simulink model "VB_RI_EKF_GNSS_INS25"  (R2023a)
settings: Solver=FixedStepAuto  StartTime=0  StopTime=200  FixedStep=0.01  RelTol=1e-3
InitFcn:
  | %resilient_initNavigation1216;
  | %init_param;
values from neighbouring files (symbols this model uses):
  C = zeros(n,m)    [utchol.m]
undefined symbols (not defined in the file or in its folder): dt, dtDelay, g0, gam0_rad, GNSSoutragetime, ISUS_flag, magnitude, p, P0, P0_RIEKF, param, pd0, pe0, phi0_rad, pn0, psi, psi0_rad, state_dim, vd0, ve0, vn0
libraries: simulink_extras x133, simulink x81, dspstat3 x81, sharedtransform x69, sharedTrackingLibrary x17, matrix_library x15, deeplib x6, dspfactors x4, aerolibconvert2 x4, aerolibtransform2 x4, dspsrcs4 x1
(part 24 of 32)

== system VB_RI_EKF_GNSS_INS25/ISUS_RIEKF3/Error State Kalman Filter M2/Extended Kalman Filter M1/Predict/If Action Subsystem ==
  Action Port : ActionPort
  Constant : Constant  Value=0
  Data Store Read : DataStoreRead  DataStoreName=x  IndexOptions=Index vector (dialog)  Indices=1  OutputSizes=1
  Data Store Write : DataStoreWrite  DataStoreName=x  IndexOptions=Index vector (dialog)  Indices=1  OutputSizes=1
  Data Store Write1 : DataStoreWrite  DataStoreName=feedback_flag_18dim  IndexOptions=Index vector (dialog)  Indices=1  OutputSizes=1
  Mux : Mux  Inputs=2
  Selector : Selector  InputPortWidth=18  IndexOptions=Index vector (dialog)  Indices=[16 17 18]  OutputSizes=1
  Zero : Constant  Value=zeros(15,1)  OutDataTypeStr=Inherit: Inherit via back propagation
  wires:
  Mux/1 -> Data Store Write/1
  Selector/1 -> Mux/2
  Zero/1 -> Mux/1
  Data Store Read/1 -> Selector/1
  Constant/1 -> Data Store Write1/1

== system VB_RI_EKF_GNSS_INS25/ISUS_RIEKF3/Error State Kalman Filter M2/bak/Simulink Function - State Transition Jacobian/Cal Phi1 ==
  Rbn : Inport
  vn : Inport  Port=2
  pn : Inport  Port=3
  Constant : Constant  Value=dt
  MATLAB Function1 : MATLAB Function  TreatAsAtomicUnit=on
  Reshape : Reshape  OutputDimensionality=Column vector (2-D)
  Reshape1 : Reshape  OutputDimensionality=Column vector (2-D)
  Phi : Outport
  wires:
  Constant/1 -> MATLAB Function1/4(dt)
  MATLAB Function1/1(Phi) -> Phi/1
  Rbn/1 -> MATLAB Function1/3(Rbn)
  vn/1 -> Reshape/1
  pn/1 -> Reshape1/1
  Reshape/1 -> MATLAB Function1/1(vn)
  Reshape1/1 -> MATLAB Function1/2(pn)

== system VB_RI_EKF_GNSS_INS25/ISUS_RIEKF3/Error State Kalman Filter M3/Extended Kalman Filter M1/Correct M1/Subsystem2 ==
  Pk_1_ISIU : Inport
  Pk_2 : Inport  Port=2
  Constant : Constant  Value=ISUS_flag
  Data Type Conversion : DataTypeConversion  OutDataTypeStr=single  SaturateOnIntegerOverflow=off  RndMeth=Floor
  MATLAB Function1 : MATLAB Function  TreatAsAtomicUnit=on
  y1 : Outport
  wires:
  MATLAB Function1/1(y) -> y1/1
  Pk_1_ISIU/1 -> Data Type Conversion/1
  Pk_2/1 -> MATLAB Function1/2(X)
  Constant/1 -> MATLAB Function1/3(ISUS_flag)
  Data Type Conversion/1 -> MATLAB Function1/1(u)

== system VB_RI_EKF_GNSS_INS25/ISUS_RIEKF3/Error State Kalman Filter M3/Extended Kalman Filter M1/Correct M1/innovation calculation1 ==
  Pk/k_1 : Inport
  yMeas : Inport  Port=2
  X : Inport  Port=3
  R : Inport  Port=4
  H : Inport  Port=5
  beta_k : Inport  Port=6
  Rk1 : Inport  Port=7
  Add : Sum
  Add1 : Sum  Inputs=+-
  Cast To Double1 : DataTypeConversion  OutDataTypeStr=single  SaturateOnIntegerOverflow=off  RndMeth=Floor
  Cast To Double2 : DataTypeConversion  OutDataTypeStr=single  SaturateOnIntegerOverflow=off  RndMeth=Floor
  Constant : Constant  Value=1/3  OutDataTypeStr=single
  Delay : Delay  DelayLength=1  InitialConditionSource=Input port
      settings: InputPortMap=u0,p4
  MATLAB Function : MATLAB Function  TreatAsAtomicUnit=on
  MATLAB Function1 : MATLAB Function  TreatAsAtomicUnit=on
  MATLAB Function2 : MATLAB Function  TreatAsAtomicUnit=on
  MATLAB Function4 : MATLAB Function  Commented=on  TreatAsAtomicUnit=on
  Product : Product  Inputs=3  Multiplication=Matrix(*)
  Product1 : Product  Multiplication=Matrix(*)
  Product2 : Product  Multiplication=Matrix(*)
  Scope1 : Scope
  Scope2 : Scope
  Transpose : Math  Operator=transpose
  Transpose1 : Math  Operator=transpose
  Sk : Outport
  m_innov : Outport  Port=2
  beta : Outport  Port=3
  R_k : Outport  Port=4
  wires:
  MATLAB Function/1(y) -> Product/2
  Product/1 -> Add/1
  Transpose/1 -> Product/3
  R/1 -> MATLAB Function2/2(R)
  Pk/k_1/1 -> MATLAB Function/1(u)
  yMeas/1 -> Add1/1
  H/1 -> Product1/1, Product/1, Transpose/1
  X/1 -> Product1/2, Scope2/1
  Product1/1 -> Add1/2
  Add/1 -> Cast To Double1/1  "S"
  Add1/1 -> Product2/2, Transpose1/1, m_innov/1, Scope1/1
  Transpose1/1 -> Product2/1
  MATLAB Function2/1(R_k) -> Cast To Double2/1
  beta_k/1 -> Delay/1
  Constant/1 -> Delay/2
  Delay/1 -> MATLAB Function2/1(beta_k)
  MATLAB Function1/1(beta) -> beta/1
  Cast To Double1/1 -> MATLAB Function1/2(S), Sk/1
  Cast To Double2/1 -> R_k/1
  Rk1/1 -> Add/2
  Product2/1 -> MATLAB Function1/1(r)

== system VB_RI_EKF_GNSS_INS25/ISUS_RIEKF3/Error State Kalman Filter M3/Extended Kalman Filter M1/Predict/If Action Subsystem ==
  Action Port : ActionPort
  Constant : Constant  Value=0
  Data Store Read : DataStoreRead  DataStoreName=x  IndexOptions=Index vector (dialog)  Indices=1  OutputSizes=1
  Data Store Write : DataStoreWrite  DataStoreName=x  IndexOptions=Index vector (dialog)  Indices=1  OutputSizes=1
  Data Store Write1 : DataStoreWrite  DataStoreName=feedback_flag_18dim  IndexOptions=Index vector (dialog)  Indices=1  OutputSizes=1
  Mux : Mux  Inputs=2
  Selector : Selector  InputPortWidth=18  IndexOptions=Index vector (dialog)  Indices=[16 17 18]  OutputSizes=1
  Zero : Constant  Value=zeros(15,1)  OutDataTypeStr=Inherit: Inherit via back propagation
  wires:
  Constant/1 -> Data Store Write1/1
  Data Store Read/1 -> Selector/1
  Zero/1 -> Mux/1
  Selector/1 -> Mux/2
  Mux/1 -> Data Store Write/1

== system VB_RI_EKF_GNSS_INS25/ISUS_RIEKF3/Error State Kalman Filter M3/bak/Simulink Function - State Transition Jacobian/Cal Phi1 ==
  Rbn : Inport
  vn : Inport  Port=2
  pn : Inport  Port=3
  Constant : Constant  Value=dt
  MATLAB Function1 : MATLAB Function  TreatAsAtomicUnit=on
  Reshape : Reshape  OutputDimensionality=Column vector (2-D)
  Reshape1 : Reshape  OutputDimensionality=Column vector (2-D)
  Phi : Outport
  wires:
  Reshape1/1 -> MATLAB Function1/2(pn)
  Reshape/1 -> MATLAB Function1/1(vn)
  pn/1 -> Reshape1/1
  vn/1 -> Reshape/1
  Rbn/1 -> MATLAB Function1/3(Rbn)
  MATLAB Function1/1(Phi) -> Phi/1
  Constant/1 -> MATLAB Function1/4(dt)

== system VB_RI_EKF_GNSS_INS25/ISUS_RIEKF3/INS propogation/Init_PVQ/Horizontal_attitude/Deal with zero ==
  In1 : Inport
  Add5 : Sum
  Constant1 : Constant  Value=1e-6  OutDataTypeStr=single
  Out1 : Outport
  wires:
  Constant1/1 -> Add5/2
  In1/1 -> Add5/1
  Add5/1 -> Out1/1

== system VB_RI_EKF_GNSS_INS25/ISUS_RIEKF3/INS propogation/gyro bias compensation/error compensation/If Action Subsystem1 ==
  Action Port : ActionPort  ActionPortLabel=if(u1 == 1)
  Constant : Constant
  Data Store Write : DataStoreWrite  DataStoreName=feedback_flag_18dim_RIEKF  IndexOptions=Index vector (dialog)  Indices=1  OutputSizes=1
  wires:
  Constant/1 -> Data Store Write/1

== system VB_RI_EKF_GNSS_INS25/ISUS_RIEKF3/INS propogation1/Init_PVQ/Horizontal_attitude/Deal with zero ==
  In1 : Inport
  Add5 : Sum
  Constant1 : Constant  Value=1e-6  OutDataTypeStr=single
  Out1 : Outport
  wires:
  Add5/1 -> Out1/1
  In1/1 -> Add5/1
  Constant1/1 -> Add5/2

== system VB_RI_EKF_GNSS_INS25/ISUS_RIEKF3/INS propogation1/gyro bias compensation/error compensation/If Action Subsystem1 ==
  Action Port : ActionPort  ActionPortLabel=if(u1 == 1)
  Constant : Constant
  Data Store Write : DataStoreWrite  DataStoreName=feedback_flag_18dim_RIEKF  IndexOptions=Index vector (dialog)  Indices=1  OutputSizes=1
  wires:
  Constant/1 -> Data Store Write/1

== system VB_RI_EKF_GNSS_INS25/ISUS_RIEKF3/INS propogation2/Init_PVQ/Horizontal_attitude/Deal with zero ==
  In1 : Inport
  Add5 : Sum
  Constant1 : Constant  Value=1e-6  OutDataTypeStr=single
  Out1 : Outport
  wires:
  Constant1/1 -> Add5/2
  In1/1 -> Add5/1
  Add5/1 -> Out1/1

== system VB_RI_EKF_GNSS_INS25/ISUS_RIEKF3/INS propogation2/gyro bias compensation/error compensation/If Action Subsystem1 ==
  Action Port : ActionPort  ActionPortLabel=if(u1 == 1)
  Constant : Constant
  Data Store Write : DataStoreWrite  DataStoreName=feedback_flag_18dim_RIEKF  IndexOptions=Index vector (dialog)  Indices=1  OutputSizes=1
  wires:
  Constant/1 -> Data Store Write/1

== system VB_RI_EKF_GNSS_INS25/ISUS_RIEKF3/INS propogation3/Init_PVQ/Horizontal_attitude/Deal with zero ==
  In1 : Inport
  Add5 : Sum
  Constant1 : Constant  Value=1e-6  OutDataTypeStr=single
  Out1 : Outport
  wires:
  Add5/1 -> Out1/1
  In1/1 -> Add5/1
  Constant1/1 -> Add5/2

== system VB_RI_EKF_GNSS_INS25/ISUS_RIEKF3/INS propogation3/gyro bias compensation/error compensation/If Action Subsystem1 ==
  Action Port : ActionPort  ActionPortLabel=if(u1 == 1)
  Constant : Constant
  Data Store Write : DataStoreWrite  DataStoreName=feedback_flag_18dim_RIEKF  IndexOptions=Index vector (dialog)  Indices=1  OutputSizes=1
  wires:
  Constant/1 -> Data Store Write/1

== system VB_RI_EKF_GNSS_INS25/RI EKF_AOA_LSTM/Error State Kalman Filter/Extended Kalman Filter1/Correct1/IGG_check ==
  Pk/k_1 : Inport
  yMeas : Inport  Port=2
  X : Inport  Port=3
  R : Inport  Port=4
  Abs : Abs  Commented=on  SaturateOnIntegerOverflow=off
  Abs1 : Abs  Commented=on  SaturateOnIntegerOverflow=off
  Add : Sum  Commented=on
  Add1 : Sum  Inputs=+-
  Add2 : Sum  Commented=on
  Constant : Constant  Commented=on  Value=12
  Constant1 : Constant  Commented=on  Value=8
  Constant2 : Constant  Value=25
  Constant3 : Constant  Commented=on  Value=eps
  Constant4 : Constant  Commented=on  Value=15
  Constant6 : Constant  Value=[zeros(6,3),eye(6),zeros(6,6)]  OutDataTypeStr=single
  Divide : Product  Commented=on  Inputs=*/
  Extract Diagonal1 : matrix_library/Extract Diagonal  Commented=on
  MATLAB Function : MATLAB Function  Commented=on  TreatAsAtomicUnit=on
  Product : Product  Inputs=3  Multiplication=Matrix(*)
  Product1 : Product  Multiplication=Matrix(*)
  Product2 : Product
  Scope : Scope  Commented=on
  Sqrt1 : Sqrt  Commented=on
  Transpose : Math  Operator=transpose
  yMeas1 : InportShadow  Port=2
  yMeas_out : Outport
  w : Outport  Port=2
  inno : Outport  Port=3
  wires:
  Product/1 -> Add/1
  Transpose/1 -> Product/3
  R/1 -> Add/2
  Pk/k_1/1 -> Product/2
  yMeas/1 -> Add1/1
  Constant6/1 -> Product1/1, Product/1, Transpose/1
  X/1 -> Product1/2
  Product1/1 -> Add1/2
  Product2/1 -> yMeas_out/1
  Add/1 -> Extract Diagonal1/1  "S"
  Divide/1 -> Abs/1, Scope/1
  MATLAB Function/1(w) -> w/1, Product2/1
  Extract Diagonal1/1 -> Abs1/1
  Add1/1 -> inno/1, Divide/1
  Sqrt1/1 -> Add2/1
  Abs/1 -> MATLAB Function/1(err)
  Abs1/1 -> Sqrt1/1
  Add2/1 -> Divide/2
  Constant3/1 -> Add2/2
  yMeas1/1 -> Product2/2
  Constant1/1 -> MATLAB Function/2(k0)
  Constant4/1 -> MATLAB Function/3(k1)
  Constant/1 -> MATLAB Function/4(zk0)
  Constant2/1 -> MATLAB Function/5(zk1)

== system VB_RI_EKF_GNSS_INS25/RI EKF_AOA_LSTM/Error State Kalman Filter/Extended Kalman Filter1/Predict/If Action Subsystem ==
  Action Port : ActionPort
  Constant : Constant  Value=0
  Data Store Read : DataStoreRead  DataStoreName=x  IndexOptions=Index vector (dialog)  Indices=1  OutputSizes=1
  Data Store Write : DataStoreWrite  DataStoreName=x  IndexOptions=Index vector (dialog)  Indices=1  OutputSizes=1
  Data Store Write1 : DataStoreWrite  DataStoreName=feedback_flag_18dim  IndexOptions=Index vector (dialog)  Indices=1  OutputSizes=1
  Mux : Mux  Inputs=2
  Selector : Selector  InputPortWidth=18  IndexOptions=Index vector (dialog)  Indices=[16 17 18]  OutputSizes=1
  Zero : Constant  Value=zeros(15,1)  OutDataTypeStr=Inherit: Inherit via back propagation
  wires:
  Mux/1 -> Data Store Write/1
  Selector/1 -> Mux/2
  Zero/1 -> Mux/1
  Data Store Read/1 -> Selector/1
  Constant/1 -> Data Store Write1/1

== system VB_RI_EKF_GNSS_INS25/RI EKF_AOA_LSTM/Error State Kalman Filter/bak/Simulink Function - State Transition Jacobian/Cal Phi1 ==
  Rbn : Inport
  vn : Inport  Port=2
  pn : Inport  Port=3
  Constant : Constant  Value=dt
  MATLAB Function1 : MATLAB Function  TreatAsAtomicUnit=on
  Reshape : Reshape  OutputDimensionality=Column vector (2-D)
  Reshape1 : Reshape  OutputDimensionality=Column vector (2-D)
  Phi : Outport
  wires:
  Constant/1 -> MATLAB Function1/4(dt)
  MATLAB Function1/1(Phi) -> Phi/1
  Rbn/1 -> MATLAB Function1/3(Rbn)
  vn/1 -> Reshape/1
  pn/1 -> Reshape1/1
  Reshape/1 -> MATLAB Function1/1(vn)
  Reshape1/1 -> MATLAB Function1/2(pn)

== system VB_RI_EKF_GNSS_INS25/RI EKF_AOA_LSTM/INS propogation/AOA//SA//Vwind update/Subsystem/Subsystem ==
  In1 : Inport
  v : Inport  Port=2
  Asin : Trigonometry  Operator=asin
  Math Function : Math  Operator=magnitude^2
  Product1 : Product
  Reciprocal Sqrt : Sqrt  Operator=rSqrt
  Sum of Elements : Sum  Inputs=+
  beta : Outport
  wires:
  Product1/1 -> Asin/1
  Sum of Elements/1 -> Reciprocal Sqrt/1
  Math Function/1 -> Sum of Elements/1
  Reciprocal Sqrt/1 -> Product1/1
  Asin/1 -> beta/1  "beta"
  In1/1 -> Math Function/1
  v/1 -> Product1/2

== system VB_RI_EKF_GNSS_INS25/RI EKF_AOA_LSTM/INS propogation/AOA//SA//Vwind update/Subsystem/Subsystem1 ==
  gyro_raw : Inport
  elevator_aileron_rudder_deg : Inport  Port=2
  accl_raw : Inport  Port=3
  TAS : Inport  Port=4
  Enable : EnablePort
  Compare To Constant : simulink/Logic and Bit Operations/Compare To Constant  relop===  const=9  OutDataTypeStr=boolean
  Counter Limited : simulink/Sources/Counter Limited  uplimit=9  tsamp=-1
  Data Type Conversion5 : DataTypeConversion  OutDataTypeStr=single  SaturateOnIntegerOverflow=off  RndMeth=Floor
  Degrees to Radians{,1..5} (6 alike) : simulink_extras/Transformations/Degrees to Radians
  LSTM predict : Subsystem
  LSTM predict1 : Subsystem
  MATLAB Function1 : MATLAB Function  TreatAsAtomicUnit=on
  MATLAB Function3 : MATLAB Function  TreatAsAtomicUnit=on
  MATLAB Function4 : MATLAB Function  Commented=on  TreatAsAtomicUnit=on
  Memory : Memory
  Memory1 : Memory
  Moving Average1 : dspstat3/Moving Average  Method=Sliding window  ForgettingFactorPort=off  SpecifyWindowLength=on  WindowLength=4  OverlapLength=3  AllowArbitraryInputLength=off  ForgettingFactor=0.9  SimulateUsing=Code generation
  Mux : Mux  Inputs=3
  Mux1 : Mux
  Radians to Degrees5 : simulink_extras/Transformations/Radians to Degrees  Commented=on
  Scope : Scope
  Selector : Selector  InputPortWidth=3  IndexOptions=Index vector (dialog)  Indices=[2]  OutputSizes=1
  Selector{1..3,5} (4 alike) : Selector  InputPortWidth=3  IndexOptions=Index vector (dialog)  Indices=[1]  OutputSizes=1
  Selector4 : Selector  InputPortWidth=3  IndexOptions=Index vector (dialog)  Indices=[3]  OutputSizes=1
  Selector6 : Selector  InputPortWidth=3  IndexOptions=Index vector (dialog)  Indices=[3]  OutputSizes=1
  TAS_1 : InportShadow  Port=4
  az : InportShadow  Port=3
  elevator_aileron_rudder_deg_1 : InportShadow  Port=2
  gyro_raw_1 : InportShadow
  AOA_LSTM_rad out : Outport
  SA_LSTM_rad : Outport  Port=2
  wires:
  elevator_aileron_rudder_deg_1/1 -> Selector6/1
  TAS/1 -> Selector2/1
  gyro_raw/1 -> Selector/1
  Degrees to Radians5/1 -> SA_LSTM_rad/1
  Degrees to Radians/1 -> Mux/3
  Selector1/1 -> Degrees to Radians/1
  Memory1/1 -> MATLAB Function3/4(beta)
  MATLAB Function1/1(Cl) -> Data Type Conversion5/1
  accl_raw/1 -> MATLAB Function1/1(axyz)
  Mux/1 -> LSTM predict/1(X), MATLAB Function4/1(u)
  MATLAB Function3/1(Cy) -> Mux1/2
  Selector/1 -> Mux/1
  Selector2/1 -> MATLAB Function1/2(TAS)  "|TAS|"
  LSTM predict1/1(YPred_test_out) -> Degrees to Radians3/1, Degrees to Radians5/1  "LSTM_SA"
  Degrees to Radians3/1 -> Memory1/1
  Degrees to Radians2/1 -> Memory/1
  Degrees to Radians1/1 -> Mux1/3
  az/1 -> MATLAB Function3/1(axyz)
  Selector5/1 -> MATLAB Function3/2(TAS)  "|TAS|"
  TAS_1/1 -> Selector5/1
  LSTM predict/1(YPred_test_out) -> Moving Average1/1, Degrees to Radians4/1
  Degrees to Radians4/1 -> AOA_LSTM_rad out/1
  elevator_aileron_rudder_deg/1 -> Selector1/1
  Memory/1 -> MATLAB Function3/3(alpha), MATLAB Function1/3(alpha)
  Data Type Conversion5/1 -> Mux/2
  Selector6/1 -> Degrees to Radians1/1
  MATLAB Function4/1(CalculatedAttackAngleFiltered) -> Radians to Degrees5/1
  Mux1/1 -> LSTM predict1/1(X)
  Moving Average1/1 -> Degrees to Radians2/1  "LSTM_AOA"
  gyro_raw_1/1 -> Selector3/1, Selector4/1
  Selector3/1 -> Mux1/1
  Selector4/1 -> Mux1/4
  Compare To Constant/1 -> LSTM predict1/Enable, LSTM predict/Enable
  Counter Limited/1 -> Scope/1, Compare To Constant/1

== system VB_RI_EKF_GNSS_INS25/RI EKF_AOA_LSTM/INS propogation/AOA//SA//Vwind update/Subsystem/Subsystem2 ==
  In1 : Inport
  v : Inport  Port=2
  Asin : Trigonometry  Operator=asin
  Math Function : Math  Operator=magnitude^2
  Product1 : Product
  Reciprocal Sqrt : Sqrt  Operator=rSqrt
  Sum of Elements : Sum  Inputs=+
  beta : Outport
  wires:
  v/1 -> Product1/2
  In1/1 -> Math Function/1
  Asin/1 -> beta/1  "beta"
  Reciprocal Sqrt/1 -> Product1/1
  Math Function/1 -> Sum of Elements/1
  Sum of Elements/1 -> Reciprocal Sqrt/1
  Product1/1 -> Asin/1

== system VB_RI_EKF_GNSS_INS25/RI EKF_AOA_LSTM/INS propogation/Init_PVQ/Horizontal_attitude/Deal with zero ==
  In1 : Inport
  Add5 : Sum
  Constant1 : Constant  Value=1e-6  OutDataTypeStr=single
  Out1 : Outport
  wires:
  Add5/1 -> Out1/1
  In1/1 -> Add5/1
  Constant1/1 -> Add5/2

== system VB_RI_EKF_GNSS_INS25/RI EKF_AOA_LSTM/INS propogation/gyro bias compensation/error compensation/If Action Subsystem1 ==
  Action Port : ActionPort  ActionPortLabel=if(u1 == 1)
  Constant : Constant
  Data Store Write : DataStoreWrite  DataStoreName=feedback_flag_18dim_RIEKF  IndexOptions=Index vector (dialog)  Indices=1  OutputSizes=1
  wires:
  Constant/1 -> Data Store Write/1

== system VB_RI_EKF_GNSS_INS25/RI EKF_AOA_direct1/Error State Kalman Filter/Extended Kalman Filter1/Correct1/IGG_check ==
  Pk/k_1 : Inport
  yMeas : Inport  Port=2
  X : Inport  Port=3
  R : Inport  Port=4
  Abs : Abs  Commented=on  SaturateOnIntegerOverflow=off
  Abs1 : Abs  Commented=on  SaturateOnIntegerOverflow=off
  Add : Sum  Commented=on
  Add1 : Sum  Inputs=+-
  Add2 : Sum  Commented=on
  Constant : Constant  Commented=on  Value=12
  Constant1 : Constant  Commented=on  Value=8
  Constant2 : Constant  Value=25
  Constant3 : Constant  Commented=on  Value=eps
  Constant4 : Constant  Commented=on  Value=15
  Constant6 : Constant  Value=[zeros(6,3),eye(6),zeros(6,6)]  OutDataTypeStr=single
  Divide : Product  Commented=on  Inputs=*/
  Extract Diagonal1 : matrix_library/Extract Diagonal  Commented=on
  MATLAB Function : MATLAB Function  Commented=on  TreatAsAtomicUnit=on
  Product : Product  Inputs=3  Multiplication=Matrix(*)
  Product1 : Product  Multiplication=Matrix(*)
  Product2 : Product
  Scope : Scope  Commented=on
  Sqrt1 : Sqrt  Commented=on
  Transpose : Math  Operator=transpose
  yMeas1 : InportShadow  Port=2
  yMeas_out : Outport
  w : Outport  Port=2
  inno : Outport  Port=3
  wires:
  Product/1 -> Add/1
  Transpose/1 -> Product/3
  R/1 -> Add/2
  Pk/k_1/1 -> Product/2
  yMeas/1 -> Add1/1
  Constant6/1 -> Product1/1, Product/1, Transpose/1
  X/1 -> Product1/2
  Product1/1 -> Add1/2
  Product2/1 -> yMeas_out/1
  Add/1 -> Extract Diagonal1/1  "S"
  Divide/1 -> Abs/1, Scope/1
  MATLAB Function/1(w) -> w/1, Product2/1
  Extract Diagonal1/1 -> Abs1/1
  Add1/1 -> inno/1, Divide/1
  Sqrt1/1 -> Add2/1
  Abs/1 -> MATLAB Function/1(err)
  Abs1/1 -> Sqrt1/1
  Add2/1 -> Divide/2
  Constant3/1 -> Add2/2
  yMeas1/1 -> Product2/2
  Constant1/1 -> MATLAB Function/2(k0)
  Constant4/1 -> MATLAB Function/3(k1)
  Constant/1 -> MATLAB Function/4(zk0)
  Constant2/1 -> MATLAB Function/5(zk1)

== system VB_RI_EKF_GNSS_INS25/RI EKF_AOA_direct1/Error State Kalman Filter/Extended Kalman Filter1/Predict/If Action Subsystem ==
  Action Port : ActionPort
  Constant : Constant  Value=0
  Data Store Read : DataStoreRead  DataStoreName=x  IndexOptions=Index vector (dialog)  Indices=1  OutputSizes=1
  Data Store Write : DataStoreWrite  DataStoreName=x  IndexOptions=Index vector (dialog)  Indices=1  OutputSizes=1
  Data Store Write1 : DataStoreWrite  DataStoreName=feedback_flag_18dim  IndexOptions=Index vector (dialog)  Indices=1  OutputSizes=1
  Mux : Mux  Inputs=2
  Selector : Selector  InputPortWidth=18  IndexOptions=Index vector (dialog)  Indices=[16 17 18]  OutputSizes=1
  Zero : Constant  Value=zeros(15,1)  OutDataTypeStr=Inherit: Inherit via back propagation
  wires:
  Mux/1 -> Data Store Write/1
  Selector/1 -> Mux/2
  Zero/1 -> Mux/1
  Data Store Read/1 -> Selector/1
  Constant/1 -> Data Store Write1/1

== system VB_RI_EKF_GNSS_INS25/RI EKF_AOA_direct1/Error State Kalman Filter/bak/Simulink Function - State Transition Jacobian/Cal Phi1 ==
  Rbn : Inport
  vn : Inport  Port=2
  pn : Inport  Port=3
  Constant : Constant  Value=dt
  MATLAB Function1 : MATLAB Function  TreatAsAtomicUnit=on
  Reshape : Reshape  OutputDimensionality=Column vector (2-D)
  Reshape1 : Reshape  OutputDimensionality=Column vector (2-D)
  Phi : Outport
  wires:
  Constant/1 -> MATLAB Function1/4(dt)
  MATLAB Function1/1(Phi) -> Phi/1
  Rbn/1 -> MATLAB Function1/3(Rbn)
  vn/1 -> Reshape/1
  pn/1 -> Reshape1/1
  Reshape/1 -> MATLAB Function1/1(vn)
  Reshape1/1 -> MATLAB Function1/2(pn)

== system VB_RI_EKF_GNSS_INS25/RI EKF_AOA_direct1/INS propogation/AOA//SA//Vwind update/Subsystem/Subsystem ==
  In1 : Inport
  v : Inport  Port=2
  Asin : Trigonometry  Operator=asin
  Math Function : Math  Operator=magnitude^2
  Product1 : Product
  Reciprocal Sqrt : Sqrt  Operator=rSqrt
  Sum of Elements : Sum  Inputs=+
  beta : Outport
  wires:
  Product1/1 -> Asin/1
  Sum of Elements/1 -> Reciprocal Sqrt/1
  Math Function/1 -> Sum of Elements/1
  Reciprocal Sqrt/1 -> Product1/1
  Asin/1 -> beta/1  "beta"
  In1/1 -> Math Function/1
  v/1 -> Product1/2

== system VB_RI_EKF_GNSS_INS25/RI EKF_AOA_direct1/INS propogation/AOA//SA//Vwind update/Subsystem/Subsystem1 ==
  gyro_raw : Inport
  elevator_aileron_rudder_deg : Inport  Port=2
  accl_raw : Inport  Port=3
  TAS : Inport  Port=4
  Enable : EnablePort
  Data Type Conversion5 : DataTypeConversion  OutDataTypeStr=single  SaturateOnIntegerOverflow=off  RndMeth=Floor
  Degrees to Radians{,1..5} (6 alike) : simulink_extras/Transformations/Degrees to Radians
  LSTM predict : Subsystem
  LSTM predict1 : Subsystem
  MATLAB Function1 : MATLAB Function  TreatAsAtomicUnit=on
  MATLAB Function3 : MATLAB Function  TreatAsAtomicUnit=on
  MATLAB Function4 : MATLAB Function  Commented=on  TreatAsAtomicUnit=on
  Memory : Memory
  Memory1 : Memory
  Moving Average : dspstat3/Moving Average  Method=Sliding window  ForgettingFactorPort=off  SpecifyWindowLength=on  WindowLength=4  OverlapLength=3  AllowArbitraryInputLength=off  ForgettingFactor=0.9  SimulateUsing=Code generation
  Moving Average1 : dspstat3/Moving Average  Method=Sliding window  ForgettingFactorPort=off  SpecifyWindowLength=on  WindowLength=4  OverlapLength=3  AllowArbitraryInputLength=off  ForgettingFactor=0.9  SimulateUsing=Code generation
  Mux : Mux  Inputs=3
  Mux1 : Mux
  Radians to Degrees5 : simulink_extras/Transformations/Radians to Degrees  Commented=on
  Selector : Selector  InputPortWidth=3  IndexOptions=Index vector (dialog)  Indices=[2]  OutputSizes=1
  Selector{1..3,5} (4 alike) : Selector  InputPortWidth=3  IndexOptions=Index vector (dialog)  Indices=[1]  OutputSizes=1
  Selector4 : Selector  InputPortWidth=3  IndexOptions=Index vector (dialog)  Indices=[3]  OutputSizes=1
  Selector6 : Selector  InputPortWidth=3  IndexOptions=Index vector (dialog)  Indices=[3]  OutputSizes=1
  TAS_1 : InportShadow  Port=4
  az : InportShadow  Port=3
  elevator_aileron_rudder_deg_1 : InportShadow  Port=2
  gyro_raw_1 : InportShadow
  AOA_LSTM_rad out : Outport
  SA_LSTM_rad : Outport  Port=2
  wires:
  elevator_aileron_rudder_deg_1/1 -> Selector6/1
  TAS/1 -> Selector2/1
  gyro_raw/1 -> Selector/1
  Degrees to Radians5/1 -> SA_LSTM_rad/1
  Degrees to Radians/1 -> Mux/3
  Selector1/1 -> Degrees to Radians/1
  Memory1/1 -> MATLAB Function3/4(beta)
  MATLAB Function1/1(Cl) -> Data Type Conversion5/1
  accl_raw/1 -> MATLAB Function1/1(axyz)
  gyro_raw_1/1 -> Selector3/1, Selector4/1
  Mux/1 -> LSTM predict/1(X), MATLAB Function4/1(u)
  MATLAB Function3/1(Cy) -> Mux1/2
  Selector/1 -> Mux/1
  Selector2/1 -> MATLAB Function1/2(TAS)  "|TAS|"
  Moving Average/1 -> Degrees to Radians3/1  "LSTM_SA"
  Degrees to Radians3/1 -> Memory1/1
  Degrees to Radians2/1 -> Memory/1
  Degrees to Radians1/1 -> Mux1/3
  az/1 -> MATLAB Function3/1(axyz)
  Selector5/1 -> MATLAB Function3/2(TAS)  "|TAS|"
  TAS_1/1 -> Selector5/1
  LSTM predict/1(YPred_test_out) -> Moving Average1/1, Degrees to Radians4/1
  Degrees to Radians4/1 -> AOA_LSTM_rad out/1
  LSTM predict1/1(YPred_test_out) -> Degrees to Radians5/1, Moving Average/1
  elevator_aileron_rudder_deg/1 -> Selector1/1
  Memory/1 -> MATLAB Function3/3(alpha), MATLAB Function1/3(alpha)
  Selector3/1 -> Mux1/1
  Data Type Conversion5/1 -> Mux/2
  Selector6/1 -> Degrees to Radians1/1
  MATLAB Function4/1(CalculatedAttackAngleFiltered) -> Radians to Degrees5/1
  Mux1/1 -> LSTM predict1/1(X)
  Selector4/1 -> Mux1/4
  Moving Average1/1 -> Degrees to Radians2/1  "LSTM_AOA"

== system VB_RI_EKF_GNSS_INS25/RI EKF_AOA_direct1/INS propogation/AOA//SA//Vwind update/Subsystem/Subsystem3 ==
  RIEKF_att_Deg : Inport
  vel_NED : Inport  Port=2
  psi_Deg : Inport  Port=3
  Enable : EnablePort
  Add1 : Sum  Inputs=+-
  Add2 : Sum  Inputs=+-
  Asin1 : Trigonometry  Operator=asin
  Atan2 : Trigonometry  Operator=atan2
  Divide1 : Product  Inputs=*/
  Fcn : Fcn  Expr=sqrt(u(1)^2+u(2)^2+u(3)^2)
  Gain : Gain  Gain=-1
  Radians to Degrees{1..4} (4 alike) : simulink_extras/Transformations/Radians to Degrees
  Selector1 : Selector  InputPortWidth=3  IndexOptions=Index vector (dialog)  Indices=[2]  OutputSizes=1
  Selector2 : Selector  InputPortWidth=3  IndexOptions=Index vector (dialog)  Indices=[3]  OutputSizes=1
  Selector3 : Selector  InputPortWidth=3  IndexOptions=Index vector (dialog)  Indices=[1]  OutputSizes=1
  AOA_direct_Deg : Outport
  SA_direct_Deg : Outport  Port=2
  wires:
  Radians to Degrees4/1 -> Add2/1  "theta"
  Radians to Degrees2/1 -> Add1/1  "theta"
  Add2/1 -> SA_direct_Deg/1  "SA_direct"
  Radians to Degrees1/1 -> Add2/2  "theta"
  psi_Deg/1 -> Radians to Degrees4/1
  Atan2/1 -> Radians to Degrees1/1
  Selector3/1 -> Atan2/2
  Selector1/1 -> Atan2/1
  Add1/1 -> AOA_direct_Deg/1  "AOA_direct"
  Gain/1 -> Divide1/1
  Fcn/1 -> Divide1/2
  Asin1/1 -> Radians to Degrees3/1
  vel_NED/1 -> Selector2/1, Fcn/1, Selector1/1, Selector3/1
  Selector2/1 -> Gain/1
  Divide1/1 -> Asin1/1
  Radians to Degrees3/1 -> Add1/2  "theta"
  RIEKF_att_Deg/1 -> Radians to Degrees2/1

== system VB_RI_EKF_GNSS_INS25/RI EKF_AOA_direct1/INS propogation/AOA//SA//Vwind update/Subsystem/Subsystem4 ==
  vel_NED : Inport
  Compare To Constant : simulink/Logic and Bit Operations/Compare To Constant  relop=>=  const=10  OutDataTypeStr=boolean
  Math Function : Math  Operator=magnitude^2
  Sqrt : Sqrt
  Sum of Elements : Sum  Inputs=+
  AOA_Estimation_flag : Outport
  wires:
  vel_NED/1 -> Math Function/1
  Math Function/1 -> Sum of Elements/1
  Compare To Constant/1 -> AOA_Estimation_flag/1
  Sqrt/1 -> Compare To Constant/1
  Sum of Elements/1 -> Sqrt/1

== system VB_RI_EKF_GNSS_INS25/RI EKF_AOA_direct1/INS propogation/Init_PVQ/Horizontal_attitude/Deal with zero ==
  In1 : Inport
  Add5 : Sum
  Constant1 : Constant  Value=1e-6  OutDataTypeStr=single
  Out1 : Outport
  wires:
  Add5/1 -> Out1/1
  In1/1 -> Add5/1
  Constant1/1 -> Add5/2

== system VB_RI_EKF_GNSS_INS25/RI EKF_AOA_direct1/INS propogation/gyro bias compensation/error compensation/If Action Subsystem1 ==
  Action Port : ActionPort  ActionPortLabel=if(u1 == 1)
  Constant : Constant
  Data Store Write : DataStoreWrite  DataStoreName=feedback_flag_18dim_RIEKF  IndexOptions=Index vector (dialog)  Indices=1  OutputSizes=1
  wires:
  Constant/1 -> Data Store Write/1

== system VB_RI_EKF_GNSS_INS25/RI EKF_AOA_ref/Error State Kalman Filter/Extended Kalman Filter1/Correct1/IGG_check ==
  Pk/k_1 : Inport
  yMeas : Inport  Port=2
  X : Inport  Port=3
  R : Inport  Port=4
  Abs : Abs  Commented=on  SaturateOnIntegerOverflow=off
  Abs1 : Abs  Commented=on  SaturateOnIntegerOverflow=off
  Add : Sum  Commented=on
  Add1 : Sum  Inputs=+-
  Add2 : Sum  Commented=on
  Constant : Constant  Commented=on  Value=12
  Constant1 : Constant  Commented=on  Value=8
  Constant2 : Constant  Value=25
  Constant3 : Constant  Commented=on  Value=eps
  Constant4 : Constant  Commented=on  Value=15
  Constant6 : Constant  Value=[zeros(6,3),eye(6),zeros(6,6)]  OutDataTypeStr=single
  Divide : Product  Commented=on  Inputs=*/
  Extract Diagonal1 : matrix_library/Extract Diagonal  Commented=on
  MATLAB Function : MATLAB Function  Commented=on  TreatAsAtomicUnit=on
  Product : Product  Inputs=3  Multiplication=Matrix(*)
  Product1 : Product  Multiplication=Matrix(*)
  Product2 : Product
  Scope : Scope  Commented=on
  Sqrt1 : Sqrt  Commented=on
  Transpose : Math  Operator=transpose
  yMeas1 : InportShadow  Port=2
  yMeas_out : Outport
  w : Outport  Port=2
  inno : Outport  Port=3
  wires:
  Constant2/1 -> MATLAB Function/5(zk1)
  Constant/1 -> MATLAB Function/4(zk0)
  Constant4/1 -> MATLAB Function/3(k1)
  Constant1/1 -> MATLAB Function/2(k0)
  yMeas1/1 -> Product2/2
  Constant3/1 -> Add2/2
  Add2/1 -> Divide/2
  Abs1/1 -> Sqrt1/1
  Abs/1 -> MATLAB Function/1(err)
  Sqrt1/1 -> Add2/1
  Add1/1 -> Divide/1, inno/1
  Extract Diagonal1/1 -> Abs1/1
  MATLAB Function/1(w) -> Product2/1, w/1
  Divide/1 -> Scope/1, Abs/1
  Add/1 -> Extract Diagonal1/1  "S"
  Product2/1 -> yMeas_out/1
  Product1/1 -> Add1/2
  X/1 -> Product1/2
  Constant6/1 -> Transpose/1, Product/1, Product1/1
  yMeas/1 -> Add1/1
  Pk/k_1/1 -> Product/2
  R/1 -> Add/2
  Transpose/1 -> Product/3
  Product/1 -> Add/1

== system VB_RI_EKF_GNSS_INS25/RI EKF_AOA_ref/Error State Kalman Filter/Extended Kalman Filter1/Predict/If Action Subsystem ==
  Action Port : ActionPort
  Constant : Constant  Value=0
  Data Store Read : DataStoreRead  DataStoreName=x  IndexOptions=Index vector (dialog)  Indices=1  OutputSizes=1
  Data Store Write : DataStoreWrite  DataStoreName=x  IndexOptions=Index vector (dialog)  Indices=1  OutputSizes=1
  Data Store Write1 : DataStoreWrite  DataStoreName=feedback_flag_18dim  IndexOptions=Index vector (dialog)  Indices=1  OutputSizes=1
  Mux : Mux  Inputs=2
  Selector : Selector  InputPortWidth=18  IndexOptions=Index vector (dialog)  Indices=[16 17 18]  OutputSizes=1
  Zero : Constant  Value=zeros(15,1)  OutDataTypeStr=Inherit: Inherit via back propagation
  wires:
  Constant/1 -> Data Store Write1/1
  Data Store Read/1 -> Selector/1
  Zero/1 -> Mux/1
  Selector/1 -> Mux/2
  Mux/1 -> Data Store Write/1

== system VB_RI_EKF_GNSS_INS25/RI EKF_AOA_ref/Error State Kalman Filter/bak/Simulink Function - State Transition Jacobian/Cal Phi1 ==
  Rbn : Inport
  vn : Inport  Port=2
  pn : Inport  Port=3
  Constant : Constant  Value=dt
  MATLAB Function1 : MATLAB Function  TreatAsAtomicUnit=on
  Reshape : Reshape  OutputDimensionality=Column vector (2-D)
  Reshape1 : Reshape  OutputDimensionality=Column vector (2-D)
  Phi : Outport
  wires:
  Reshape1/1 -> MATLAB Function1/2(pn)
  Reshape/1 -> MATLAB Function1/1(vn)
  pn/1 -> Reshape1/1
  vn/1 -> Reshape/1
  Rbn/1 -> MATLAB Function1/3(Rbn)
  MATLAB Function1/1(Phi) -> Phi/1
  Constant/1 -> MATLAB Function1/4(dt)

== system VB_RI_EKF_GNSS_INS25/RI EKF_AOA_ref/INS propogation/AOA//SA//Vwind update/Subsystem/Subsystem ==
  In1 : Inport
  v : Inport  Port=2
  Asin : Trigonometry  Operator=asin
  Math Function : Math  Operator=magnitude^2
  Product1 : Product
  Reciprocal Sqrt : Sqrt  Operator=rSqrt
  Sum of Elements : Sum  Inputs=+
  beta : Outport
  wires:
  v/1 -> Product1/2
  In1/1 -> Math Function/1
  Asin/1 -> beta/1  "beta"
  Reciprocal Sqrt/1 -> Product1/1
  Math Function/1 -> Sum of Elements/1
  Sum of Elements/1 -> Reciprocal Sqrt/1
  Product1/1 -> Asin/1

== system VB_RI_EKF_GNSS_INS25/RI EKF_AOA_ref/INS propogation/AOA//SA//Vwind update/Subsystem/Subsystem1 ==
  gyro_raw : Inport
  elevator_aileron_rudder_deg : Inport  Port=2
  accl_raw : Inport  Port=3
  TAS : Inport  Port=4
  Enable : EnablePort
  Data Type Conversion5 : DataTypeConversion  OutDataTypeStr=single  SaturateOnIntegerOverflow=off  RndMeth=Floor
  Degrees to Radians{,1..5} (6 alike) : simulink_extras/Transformations/Degrees to Radians
  LSTM predict : Subsystem
  LSTM predict1 : Subsystem
  MATLAB Function1 : MATLAB Function  TreatAsAtomicUnit=on
  MATLAB Function3 : MATLAB Function  TreatAsAtomicUnit=on
  MATLAB Function4 : MATLAB Function  Commented=on  TreatAsAtomicUnit=on
  Memory : Memory
  Memory1 : Memory
  Moving Average : dspstat3/Moving Average  Method=Sliding window  ForgettingFactorPort=off  SpecifyWindowLength=on  WindowLength=4  OverlapLength=3  AllowArbitraryInputLength=off  ForgettingFactor=0.9  SimulateUsing=Code generation
  Moving Average1 : dspstat3/Moving Average  Method=Sliding window  ForgettingFactorPort=off  SpecifyWindowLength=on  WindowLength=4  OverlapLength=3  AllowArbitraryInputLength=off  ForgettingFactor=0.9  SimulateUsing=Code generation
  Mux : Mux  Inputs=3
  Mux1 : Mux
  Radians to Degrees5 : simulink_extras/Transformations/Radians to Degrees  Commented=on
  Selector : Selector  InputPortWidth=3  IndexOptions=Index vector (dialog)  Indices=[2]  OutputSizes=1
  Selector{1..3,5} (4 alike) : Selector  InputPortWidth=3  IndexOptions=Index vector (dialog)  Indices=[1]  OutputSizes=1
  Selector4 : Selector  InputPortWidth=3  IndexOptions=Index vector (dialog)  Indices=[3]  OutputSizes=1
  Selector6 : Selector  InputPortWidth=3  IndexOptions=Index vector (dialog)  Indices=[3]  OutputSizes=1
  TAS_1 : InportShadow  Port=4
  az : InportShadow  Port=3
  elevator_aileron_rudder_deg_1 : InportShadow  Port=2
  gyro_raw_1 : InportShadow
  AOA_LSTM_rad out : Outport
  SA_LSTM_rad : Outport  Port=2
  wires:
  Moving Average1/1 -> Degrees to Radians2/1  "LSTM_AOA"
  Selector4/1 -> Mux1/4
  Mux1/1 -> LSTM predict1/1(X)
  MATLAB Function4/1(CalculatedAttackAngleFiltered) -> Radians to Degrees5/1
  Selector6/1 -> Degrees to Radians1/1
  Data Type Conversion5/1 -> Mux/2
  Selector3/1 -> Mux1/1
  Memory/1 -> MATLAB Function1/3(alpha), MATLAB Function3/3(alpha)
  elevator_aileron_rudder_deg/1 -> Selector1/1
  LSTM predict1/1(YPred_test_out) -> Moving Average/1, Degrees to Radians5/1
  Degrees to Radians4/1 -> AOA_LSTM_rad out/1
  LSTM predict/1(YPred_test_out) -> Degrees to Radians4/1, Moving Average1/1
  TAS_1/1 -> Selector5/1
  Selector5/1 -> MATLAB Function3/2(TAS)  "|TAS|"
  az/1 -> MATLAB Function3/1(axyz)
  Degrees to Radians1/1 -> Mux1/3
  Degrees to Radians2/1 -> Memory/1
  Degrees to Radians3/1 -> Memory1/1
  Moving Average/1 -> Degrees to Radians3/1  "LSTM_SA"
  Selector2/1 -> MATLAB Function1/2(TAS)  "|TAS|"
  Selector/1 -> Mux/1
  MATLAB Function3/1(Cy) -> Mux1/2
  Mux/1 -> MATLAB Function4/1(u), LSTM predict/1(X)
  gyro_raw_1/1 -> Selector4/1, Selector3/1
  accl_raw/1 -> MATLAB Function1/1(axyz)
  MATLAB Function1/1(Cl) -> Data Type Conversion5/1
  Memory1/1 -> MATLAB Function3/4(beta)
  Selector1/1 -> Degrees to Radians/1
  Degrees to Radians/1 -> Mux/3
  Degrees to Radians5/1 -> SA_LSTM_rad/1
  gyro_raw/1 -> Selector/1
  TAS/1 -> Selector2/1
  elevator_aileron_rudder_deg_1/1 -> Selector6/1

== system VB_RI_EKF_GNSS_INS25/RI EKF_AOA_ref/INS propogation/AOA//SA//Vwind update/Subsystem/Subsystem3 ==
  RIEKF_att_Deg : Inport
  vel_NED : Inport  Port=2
  psi_Deg : Inport  Port=3
  Enable : EnablePort
  Add1 : Sum  Inputs=+-
  Add2 : Sum  Inputs=+-
  Asin1 : Trigonometry  Operator=asin
  Atan2 : Trigonometry  Operator=atan2
  Divide1 : Product  Inputs=*/
  Fcn : Fcn  Expr=sqrt(u(1)^2+u(2)^2+u(3)^2)
  Gain : Gain  Gain=-1
  Radians to Degrees{1..4} (4 alike) : simulink_extras/Transformations/Radians to Degrees
  Selector1 : Selector  InputPortWidth=3  IndexOptions=Index vector (dialog)  Indices=[2]  OutputSizes=1
  Selector2 : Selector  InputPortWidth=3  IndexOptions=Index vector (dialog)  Indices=[3]  OutputSizes=1
  Selector3 : Selector  InputPortWidth=3  IndexOptions=Index vector (dialog)  Indices=[1]  OutputSizes=1
  AOA_direct_Deg : Outport
  SA_direct_Deg : Outport  Port=2
  wires:
  RIEKF_att_Deg/1 -> Radians to Degrees2/1
  Radians to Degrees3/1 -> Add1/2  "theta"
  Divide1/1 -> Asin1/1
  Selector2/1 -> Gain/1
  vel_NED/1 -> Selector3/1, Selector1/1, Fcn/1, Selector2/1
  Asin1/1 -> Radians to Degrees3/1
  Fcn/1 -> Divide1/2
  Gain/1 -> Divide1/1
  Add1/1 -> AOA_direct_Deg/1  "AOA_direct"
  Selector1/1 -> Atan2/1
  Selector3/1 -> Atan2/2
  Atan2/1 -> Radians to Degrees1/1
  psi_Deg/1 -> Radians to Degrees4/1
  Radians to Degrees1/1 -> Add2/2  "theta"
  Add2/1 -> SA_direct_Deg/1  "SA_direct"
  Radians to Degrees2/1 -> Add1/1  "theta"
  Radians to Degrees4/1 -> Add2/1  "theta"

== system VB_RI_EKF_GNSS_INS25/RI EKF_AOA_ref/INS propogation/AOA//SA//Vwind update/Subsystem/Subsystem4 ==
  vel_NED : Inport
  Compare To Constant : simulink/Logic and Bit Operations/Compare To Constant  relop=>=  const=10  OutDataTypeStr=boolean
  Math Function : Math  Operator=magnitude^2
  Sqrt : Sqrt
  Sum of Elements : Sum  Inputs=+
  AOA_Estimation_flag : Outport
  wires:
  Sum of Elements/1 -> Sqrt/1
  Sqrt/1 -> Compare To Constant/1
  Compare To Constant/1 -> AOA_Estimation_flag/1
  Math Function/1 -> Sum of Elements/1
  vel_NED/1 -> Math Function/1

== system VB_RI_EKF_GNSS_INS25/RI EKF_AOA_ref/INS propogation/Init_PVQ/Horizontal_attitude/Deal with zero ==
  In1 : Inport
  Add5 : Sum
  Constant1 : Constant  Value=1e-6  OutDataTypeStr=single
  Out1 : Outport
  wires:
  Constant1/1 -> Add5/2
  In1/1 -> Add5/1
  Add5/1 -> Out1/1

== system VB_RI_EKF_GNSS_INS25/RI EKF_AOA_ref/INS propogation/gyro bias compensation/error compensation/If Action Subsystem1 ==
  Action Port : ActionPort  ActionPortLabel=if(u1 == 1)
  Constant : Constant
  Data Store Write : DataStoreWrite  DataStoreName=feedback_flag_18dim_RIEKF  IndexOptions=Index vector (dialog)  Indices=1  OutputSizes=1
  wires:
  Constant/1 -> Data Store Write/1

== system VB_RI_EKF_GNSS_INS25/RI EKF_AOA_LSTM/INS propogation/AOA//SA//Vwind update/Subsystem/Subsystem1/LSTM predict ==
  X : Inport
  Enable : EnablePort
  Data Type Conversion11 : DataTypeConversion  OutDataTypeStr=double  SaturateOnIntegerOverflow=off  RndMeth=Floor
  MATLAB Function5 : MATLAB Function  TreatAsAtomicUnit=on
  MATLAB Function6 : MATLAB Function  TreatAsAtomicUnit=on
  Predict : deeplib/Predict  Network=Network from MAT-file  NetworkFunction=squeezenet  NetworkFilePath=C:\Users\18296\Desktop\lstmnet.mat  MiniBatchSize=128  InputDataFormats={'',''}  Predictions=on  Activations={}  ForceInterpretedSim=off  EnableDLNetwork=on
  Transpose2 : Math  Operator=transpose
  YPred_test_out : Outport
  wires:
  Predict/1 -> MATLAB Function6/1(YPred_test)
  Transpose2/1 -> Predict/1
  MATLAB Function6/1(YPred_test_out) -> YPred_test_out/1
  Data Type Conversion11/1 -> MATLAB Function5/1(X)
  X/1 -> Data Type Conversion11/1
  MATLAB Function5/1(X_nYPred) -> Transpose2/1

== system VB_RI_EKF_GNSS_INS25/RI EKF_AOA_LSTM/INS propogation/AOA//SA//Vwind update/Subsystem/Subsystem1/LSTM predict1 ==
  X : Inport
  Enable : EnablePort
  Data Type Conversion11 : DataTypeConversion  OutDataTypeStr=double  SaturateOnIntegerOverflow=off  RndMeth=Floor
  MATLAB Function5 : MATLAB Function  TreatAsAtomicUnit=on
  MATLAB Function6 : MATLAB Function  TreatAsAtomicUnit=on
  Predict : deeplib/Predict  Network=Network from MAT-file  NetworkFunction=squeezenet  NetworkFilePath=C:\Users\18296\Desktop\lstmnetSA0826.mat  MiniBatchSize=200  InputDataFormats={'',''}  Predictions=on  Activations={}  ForceInterpretedSim=off  EnableDLNetwork=on
  Transpose2 : Math  Operator=transpose
  YPred_test_out : Outport
  wires:
  MATLAB Function5/1(X_nYPred) -> Transpose2/1
  X/1 -> Data Type Conversion11/1
  Data Type Conversion11/1 -> MATLAB Function5/1(X)
  MATLAB Function6/1(YPred_test_out) -> YPred_test_out/1
  Transpose2/1 -> Predict/1
  Predict/1 -> MATLAB Function6/1(YPred_test)

== system VB_RI_EKF_GNSS_INS25/RI EKF_AOA_direct1/INS propogation/AOA//SA//Vwind update/Subsystem/Subsystem1/LSTM predict ==
  X : Inport
  Data Type Conversion11 : DataTypeConversion  OutDataTypeStr=double  SaturateOnIntegerOverflow=off  RndMeth=Floor
  MATLAB Function5 : MATLAB Function  TreatAsAtomicUnit=on
  MATLAB Function6 : MATLAB Function  TreatAsAtomicUnit=on
  Predict : deeplib/Predict  Network=Network from MAT-file  NetworkFunction=squeezenet  NetworkFilePath=D:\app\RIEKFModel\lstmnet.mat  MiniBatchSize=128  InputDataFormats={'',''}  Predictions=on  Activations={}  ForceInterpretedSim=off  EnableDLNetwork=on
  Transpose2 : Math  Operator=transpose
  YPred_test_out : Outport
  wires:
  Predict/1 -> MATLAB Function6/1(YPred_test)
  Transpose2/1 -> Predict/1
  MATLAB Function6/1(YPred_test_out) -> YPred_test_out/1
  Data Type Conversion11/1 -> MATLAB Function5/1(X)
  X/1 -> Data Type Conversion11/1
  MATLAB Function5/1(X_nYPred) -> Transpose2/1

== system VB_RI_EKF_GNSS_INS25/RI EKF_AOA_direct1/INS propogation/AOA//SA//Vwind update/Subsystem/Subsystem1/LSTM predict1 ==
  X : Inport
  Data Type Conversion11 : DataTypeConversion  OutDataTypeStr=double  SaturateOnIntegerOverflow=off  RndMeth=Floor
  MATLAB Function5 : MATLAB Function  TreatAsAtomicUnit=on
  MATLAB Function6 : MATLAB Function  TreatAsAtomicUnit=on
  Predict : deeplib/Predict  Network=Network from MAT-file  NetworkFunction=squeezenet  NetworkFilePath=D:\app\RIEKFModel\lstmnetSA.mat  MiniBatchSize=128  InputDataFormats={'',''}  Predictions=on  Activations={}  ForceInterpretedSim=off  EnableDLNetwork=on
  Transpose2 : Math  Operator=transpose
  YPred_test_out : Outport
  wires:
  MATLAB Function5/1(X_nYPred) -> Transpose2/1
  X/1 -> Data Type Conversion11/1
  Data Type Conversion11/1 -> MATLAB Function5/1(X)
  MATLAB Function6/1(YPred_test_out) -> YPred_test_out/1
  Transpose2/1 -> Predict/1
  Predict/1 -> MATLAB Function6/1(YPred_test)

== system VB_RI_EKF_GNSS_INS25/RI EKF_AOA_ref/INS propogation/AOA//SA//Vwind update/Subsystem/Subsystem1/LSTM predict ==
  X : Inport
  Data Type Conversion11 : DataTypeConversion  OutDataTypeStr=double  SaturateOnIntegerOverflow=off  RndMeth=Floor
  MATLAB Function5 : MATLAB Function  TreatAsAtomicUnit=on
  MATLAB Function6 : MATLAB Function  TreatAsAtomicUnit=on
  Predict : deeplib/Predict  Network=Network from MAT-file  NetworkFunction=squeezenet  NetworkFilePath=D:\app\RIEKFModel\lstmnet.mat  MiniBatchSize=128  InputDataFormats={'',''}  Predictions=on  Activations={}  ForceInterpretedSim=off  EnableDLNetwork=on
  Transpose2 : Math  Operator=transpose
  YPred_test_out : Outport
  wires:
  MATLAB Function5/1(X_nYPred) -> Transpose2/1
  X/1 -> Data Type Conversion11/1
  Data Type Conversion11/1 -> MATLAB Function5/1(X)
  MATLAB Function6/1(YPred_test_out) -> YPred_test_out/1
  Transpose2/1 -> Predict/1
  Predict/1 -> MATLAB Function6/1(YPred_test)

== system VB_RI_EKF_GNSS_INS25/RI EKF_AOA_ref/INS propogation/AOA//SA//Vwind update/Subsystem/Subsystem1/LSTM predict1 ==
  X : Inport
  Data Type Conversion11 : DataTypeConversion  OutDataTypeStr=double  SaturateOnIntegerOverflow=off  RndMeth=Floor
  MATLAB Function5 : MATLAB Function  TreatAsAtomicUnit=on
  MATLAB Function6 : MATLAB Function  TreatAsAtomicUnit=on
  Predict : deeplib/Predict  Network=Network from MAT-file  NetworkFunction=squeezenet  NetworkFilePath=D:\app\RIEKFModel\lstmnetSA.mat  MiniBatchSize=128  InputDataFormats={'',''}  Predictions=on  Activations={}  ForceInterpretedSim=off  EnableDLNetwork=on
  Transpose2 : Math  Operator=transpose
  YPred_test_out : Outport
  wires:
  Predict/1 -> MATLAB Function6/1(YPred_test)
  Transpose2/1 -> Predict/1
  MATLAB Function6/1(YPred_test_out) -> YPred_test_out/1
  Data Type Conversion11/1 -> MATLAB Function5/1(X)
  X/1 -> Data Type Conversion11/1
  MATLAB Function5/1(X_nYPred) -> Transpose2/1

== matlab function VB_RI_EKF_GNSS_INS25/ER EKF/Subsystem/MATLAB Function ==
  data: dpsi input; y output
function y = wrap_dpsi(dpsi)
    if dpsi > 180
        dpsi = dpsi -360;
    elseif dpsi < -180
        dpsi = dpsi + 360;
    else 
        dpsi = dpsi;
    end
y = dpsi;

== matlab function VB_RI_EKF_GNSS_INS25/ISUS_RIEKF3/Error State Kalman Filter M1/VB-Extended Kalman Filter M2/Correct M1/innovation calculation1/MATLAB Function3 ==
  data: r input; S input; Gamma output
function Gamma   = fcn(r, S)


Gamma = transpose(r)*inv(S)*r;

end

== matlab function VB_RI_EKF_GNSS_INS25/RI EKF_AOA_ref/Error State Kalman Filter/Cal Q1/MATLAB Function1 ==
  data: Q output; dt input
function Q = fcn(dt)
    % G.block(0, 0, 3, 3) = -exp_so3(-w_hat * dt) * Jr_so3(-w_hat * dt) * dt;
    %    G.block(6, 3, 3, 3) = -R_Gtoi.transpose() * dt;
    %    G.block(3, 3, 3, 3) = -0.5 * R_Gtoi.transpose() * dt * dt;
    %    G.block(9, 6, 3, 3).setIdentity();
    %    G.block(12, 9, 3, 3).setIdentity();
    

    cov_dim = 21;
    Q = zeros(cov_dim,cov_dim);
%     noises_sigma_a_2 = 2.0000e-4^2;
%     noises_sigma_w_2 = 1.6968e-4^2;
%     noises_sigma_ab_2 = 3.0000e-4^2;
%     noises_sigma_wb_2 = 1.9393e-5^2;
    noises_sigma_a_2 = 0.001^2*1;
    %noises_sigma_w_2 = 0.0001^2;
    noises_sigma_w_2 = 0.0001^2;
    noises_sigma_ab_2 = 1.0000e-4^2*1;
    noises_sigma_wb_2 = 0.00002^2;
    noises_sigma_mb_2 = 0.001^2;
    noises_sigma_dtheta_2 = (1/57.3)^2;
    noises_sigma_dwind_2 = 0.01^2;
    Q = diag([noises_sigma_w_2 / dt * ones(3,1); ...
                noises_sigma_a_2 / dt * ones(3,1); ...
                noises_sigma_wb_2 * dt * ones(3,1); ...
                noises_sigma_ab_2 * dt * ones(3,1); ...
                noises_sigma_mb_2 * dt * ones(3,1); ...
                noises_sigma_dtheta_2 * ones(3,1); ...
                noises_sigma_dwind_2* ones(3,1)]);
    

end
